simulink model "lab_06_02"  (R2024b)
settings: Solver=VariableStepAuto  StartTime=0.0  StopTime=10.0  RelTol=1e-3
libraries: commanapbnd3 x2
settings Model: LastModifiedBy=LENOVO

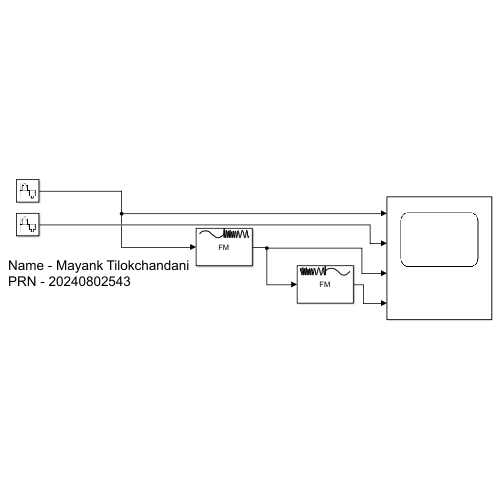
[thumbnail: Simulink's stored preview of the top-level diagram]
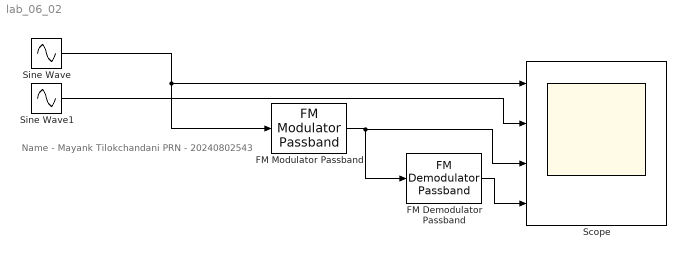
== system lab_06_02 ==
  note: Name - Mayank Tilokchandani
      | PRN - 20240802543
  FM Demodulator Passband : commanapbnd3/FM Demodulator Passband  Fc=100  Ph=0  Kc=10  Ho=100
  FM Modulator Passband : commanapbnd3/FM Modulator Passband  Fc=100  Ph=0  Kc=10
  Scope : Scope  NumInputPorts=4
  Sine Wave : Sin  Amplitude=2  Frequency=2  SampleTime=0.01
  Sine Wave1 : Sin  Amplitude=2  Frequency=20  SampleTime=0.01
  wires:
  Sine Wave/1 -> Scope/1, FM Modulator Passband/1
  Sine Wave1/1 -> Scope/2
  FM Modulator Passband/1 -> FM Demodulator Passband/1, Scope/3
  FM Demodulator Passband/1 -> Scope/4
